simulink model "Angular_Input_Sliding_Mode"  (R2022a)
settings: Solver=VariableStepAuto  StartTime=0  StopTime=tspan(2)  RelTol=1e-8
undefined symbols (not defined in the file): Angle_max, b_Sxd, b_Syd, BL_gain, K_switch, lambda_x_num, r_sim, tau_angle, Tmax, x_0
libraries: cstblocks x4
settings Model: Creator=domin  LastModifiedBy=domin
settings SolverCC: AlgebraicLoopSolver=TrustRegion
settings DataIOCC: SaveFormat=StructureWithTime
settings OptimizationCC: BlockReduction=off  BufferReuse=off
settings DebuggingCC: AlgebraicLoopMsg=none  SFMachineParentedDataDiag=warning
settings RTWCC: DLArmComputeVersion=19.05

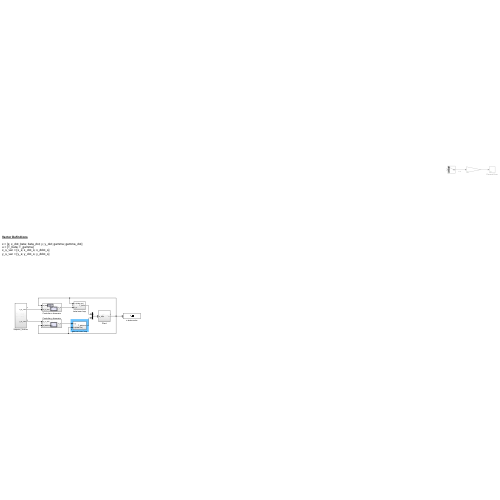
[thumbnail: Simulink's stored preview of the top-level diagram]
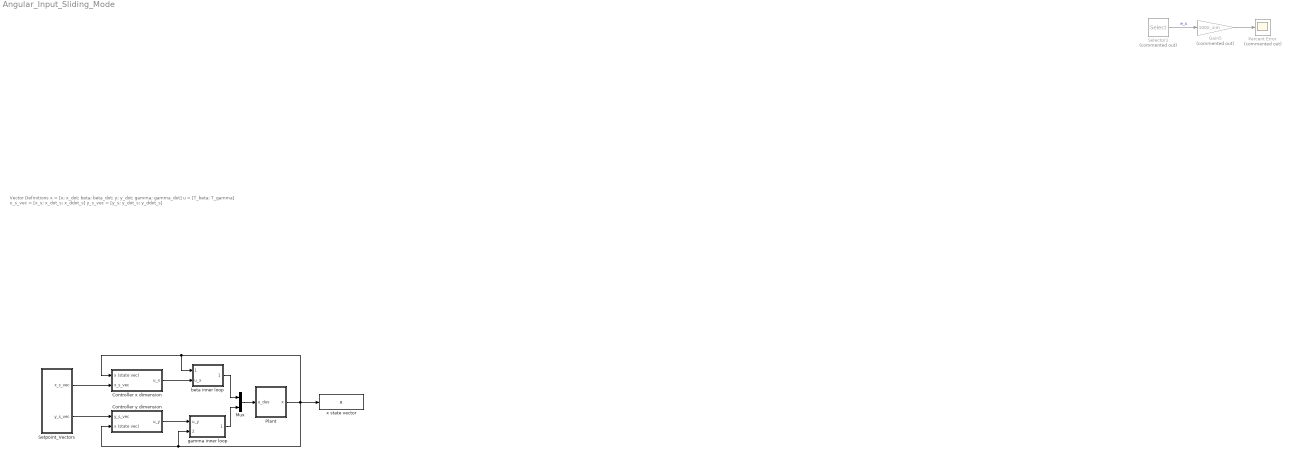
== system Angular_Input_Sliding_Mode ==
  note: Vector Definitions
      |
      | x = [x; x_dot; beta; beta_dot; y; y_dot; gamma; gamma_dot]
      | u = [T_beta; T_gamma]
      | x_s_vec = [x_s; x_dot_s; x_ddot_s]
      | y_s_vec = [y_s; y_dot_s; y_ddot_s]
  Controller x dimension : Subsystem
  Controller y dimension : Subsystem
  Gain5 : Gain  Commented=on  Gain=100/r_sim
  Mux : Mux  Inputs=2
  Percent Error : Scope  Commented=on
  Plant : Subsystem
  Selector1 : Selector  Commented=on  InputPortWidth=5  IndexOptions=Index vector (dialog)  Indices=[1]  OutputSizes=1
  Setpoint_Vectors : Subsystem
  beta inner loop : Subsystem
  gamma inner loop : Subsystem
  x state vector : ToWorkspace  VariableName=x  SampleTime=-1
  wires:
  Gain5/1 -> Percent Error/1
  Selector1/1 -> Gain5/1  "e_x"
  Controller x dimension/1(u_x) -> beta inner loop/2(u_x)
  Controller y dimension/1(u_y) -> gamma inner loop/1(u_y)
  Plant/1(x) -> Controller x dimension/1(x (state vec)), beta inner loop/1(x (state vec)), x state vector/1, Controller y dimension/2(x (state vec)), gamma inner loop/2(x (state vec))
  beta inner loop/1(T_beta) -> Mux/1
  Mux/1 -> Plant/1(u_des)
  gamma inner loop/1(T_gamma) -> Mux/2
  Setpoint_Vectors/1(x_s_vec) -> Controller x dimension/2(x_s_vec)
  Setpoint_Vectors/2(y_s_vec) -> Controller y dimension/1(y_s_vec)

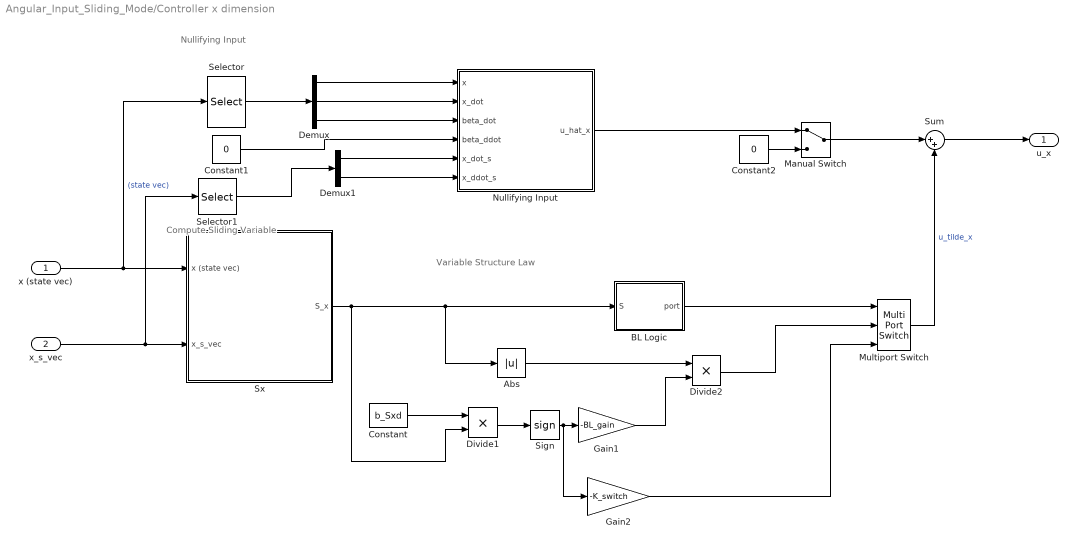
== system Angular_Input_Sliding_Mode/Controller x dimension ==
  note: Compute Sliding Variable
  note: Nullifying Input
  note: Variable Structure Law
  x (state vec) : Inport
  x_s_vec : Inport  Port=2
  Abs : Abs  SaturateOnIntegerOverflow=off
  BL Logic : MATLAB Function  TreatAsAtomicUnit=on
  Constant : Constant  Value=b_Sxd
  Constant1 : Constant  Value=0
  Constant2 : Constant  Value=0
  Demux : Demux  Outputs=3
  Demux1 : Demux  Outputs=2
  Divide1 : Product  Inputs=**
  Divide2 : Product  Inputs=**
  Gain1 : Gain  Gain=-BL_gain
  Gain2 : Gain  Gain=-K_switch
  Manual Switch : ManualSwitch
  Multiport Switch : MultiPortSwitch  Inputs=2  SaturateOnIntegerOverflow=off  InputSameDT=off
  Nullifying Input : MATLAB Function  TreatAsAtomicUnit=on
  Selector : Selector  InputPortWidth=8  IndexOptions=Index vector (dialog)  Indices=[1 2 4]  OutputSizes=1
  Selector1 : Selector  InputPortWidth=3  IndexOptions=Index vector (dialog)  Indices=[2 3]  OutputSizes=1
  Sign : Signum
  Sum : Sum  Inputs=|++
  Sx : Subsystem
  u_x : Outport
  wires:
  Sum/1 -> u_x/1
  x (state vec)/1 -> Sx/1(x (state vec)), Selector/1  "(state vec)"
  x_s_vec/1 -> Selector1/1, Sx/2(x_s_vec)
  Selector/1 -> Demux/1
  Demux/2 -> Nullifying Input/2(x_dot)
  Selector1/1 -> Demux1/1
  Demux1/1 -> Nullifying Input/5(x_dot_s)
  Demux1/2 -> Nullifying Input/6(x_ddot_s)
  Nullifying Input/1(u_hat_x) -> Manual Switch/1
  Constant/1 -> Divide1/1
  Divide2/1 -> Multiport Switch/2
  Sx/1(S_x) -> Divide1/2, Abs/1, BL Logic/1(S)
  Demux/1 -> Nullifying Input/1(x)
  Gain1/1 -> Divide2/2
  BL Logic/1(port) -> Multiport Switch/1
  Multiport Switch/1 -> Sum/2  "u_tilde_x"
  Sign/1 -> Gain2/1, Gain1/1
  Divide1/1 -> Sign/1
  Gain2/1 -> Multiport Switch/3
  Abs/1 -> Divide2/1
  Demux/3 -> Nullifying Input/3(beta_dot)
  Constant1/1 -> Nullifying Input/4(beta_ddot)
  Constant2/1 -> Manual Switch/2
  Manual Switch/1 -> Sum/1

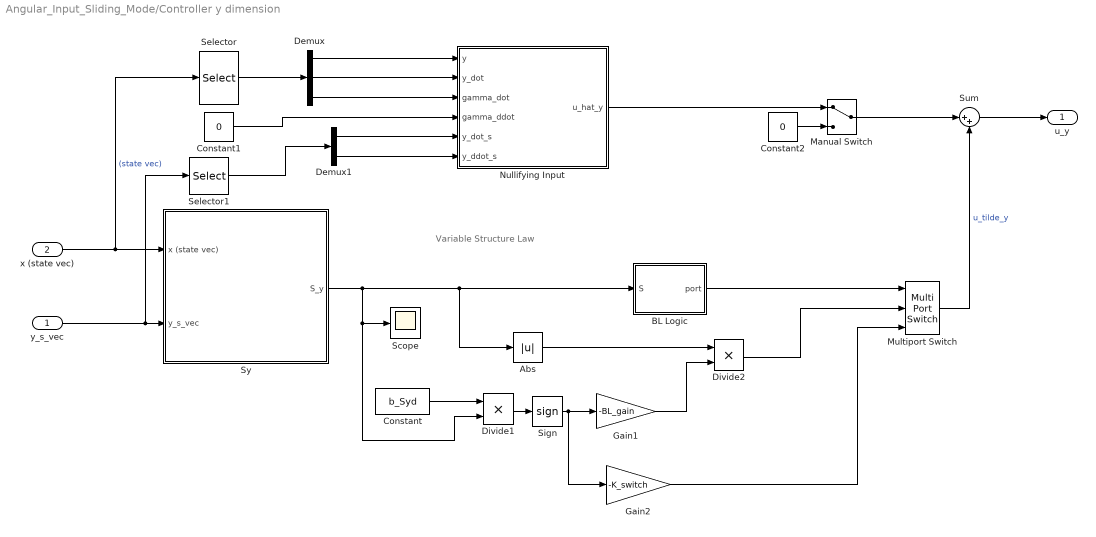
== system Angular_Input_Sliding_Mode/Controller y dimension ==
  note: Variable Structure Law
  y_s_vec : Inport
  x (state vec) : Inport  Port=2
  Abs : Abs  SaturateOnIntegerOverflow=off
  BL Logic : MATLAB Function  TreatAsAtomicUnit=on
  Constant : Constant  Value=b_Syd
  Constant1 : Constant  Value=0
  Constant2 : Constant  Value=0
  Demux : Demux  Outputs=3
  Demux1 : Demux  Outputs=2
  Divide1 : Product  Inputs=**
  Divide2 : Product  Inputs=**
  Gain1 : Gain  Gain=-BL_gain
  Gain2 : Gain  Gain=-K_switch
  Manual Switch : ManualSwitch
  Multiport Switch : MultiPortSwitch  Inputs=2  SaturateOnIntegerOverflow=off  InputSameDT=off
  Nullifying Input : MATLAB Function  TreatAsAtomicUnit=on
  Scope : Scope
  Selector : Selector  InputPortWidth=8  IndexOptions=Index vector (dialog)  Indices=[5 6 8]  OutputSizes=1
  Selector1 : Selector  InputPortWidth=3  IndexOptions=Index vector (dialog)  Indices=[2 3]  OutputSizes=1
  Sign : Signum
  Sum : Sum  Inputs=|++
  Sy : Subsystem
  u_y : Outport
  wires:
  Sum/1 -> u_y/1
  Gain1/1 -> Divide2/2
  Abs/1 -> Divide2/1
  Gain2/1 -> Multiport Switch/3
  Multiport Switch/1 -> Sum/2  "u_tilde_y"
  BL Logic/1(port) -> Multiport Switch/1
  Sign/1 -> Gain1/1, Gain2/1
  Constant/1 -> Divide1/1
  Divide2/1 -> Multiport Switch/2
  Sy/1(S_y) -> Divide1/2, Scope/1, Abs/1, BL Logic/1(S)
  Divide1/1 -> Sign/1
  Demux/3 -> Nullifying Input/3(gamma_dot)
  Demux/1 -> Nullifying Input/1(y)
  Demux1/1 -> Nullifying Input/5(y_dot_s)
  Nullifying Input/1(u_hat_y) -> Manual Switch/1
  Demux1/2 -> Nullifying Input/6(y_ddot_s)
  Selector/1 -> Demux/1
  Demux/2 -> Nullifying Input/2(y_dot)
  y_s_vec/1 -> Sy/2(y_s_vec), Selector1/1
  Selector1/1 -> Demux1/1
  x (state vec)/1 -> Sy/1(x (state vec)), Selector/1  "(state vec)"
  Constant1/1 -> Nullifying Input/4(gamma_ddot)
  Constant2/1 -> Manual Switch/2
  Manual Switch/1 -> Sum/1

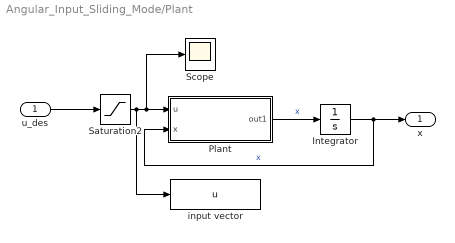
== system Angular_Input_Sliding_Mode/Plant ==
  u_des : Inport
  Integrator : Integrator  InitialCondition=x_0
  Plant : Subsystem
  Saturation2 : Saturate  UpperLimit=Tmax  LowerLimit=-Tmax  ZeroCross=off
  Scope : Scope
  input vector : ToWorkspace  VariableName=u  SampleTime=-1
  x : Outport
  wires:
  Saturation2/1 -> Scope/1, Plant/1(u), input vector/1
  Integrator/1 -> x/1, Plant/2(x)  "x"
  Plant/1(out1) -> Integrator/1  "x"
  u_des/1 -> Saturation2/1

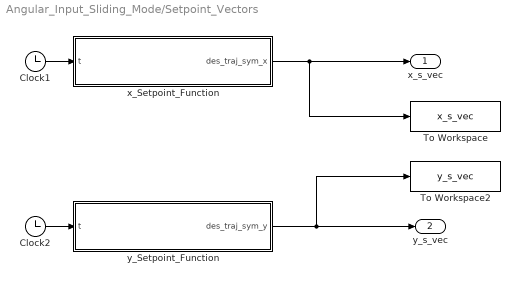
== system Angular_Input_Sliding_Mode/Setpoint_Vectors ==
  Clock1 : Clock
  Clock2 : Clock
  To Workspace : ToWorkspace  VariableName=x_s_vec  SampleTime=-1
  To Workspace2 : ToWorkspace  VariableName=y_s_vec  SampleTime=-1
  x_Setpoint_Function : MATLAB Function  TreatAsAtomicUnit=on
  y_Setpoint_Function : MATLAB Function  TreatAsAtomicUnit=on
  x_s_vec : Outport
  y_s_vec : Outport  Port=2
  wires:
  Clock2/1 -> y_Setpoint_Function/1(t)
  y_Setpoint_Function/1(des_traj_sym_y) -> y_s_vec/1, To Workspace2/1
  x_Setpoint_Function/1(des_traj_sym_x) -> x_s_vec/1, To Workspace/1
  Clock1/1 -> x_Setpoint_Function/1(t)

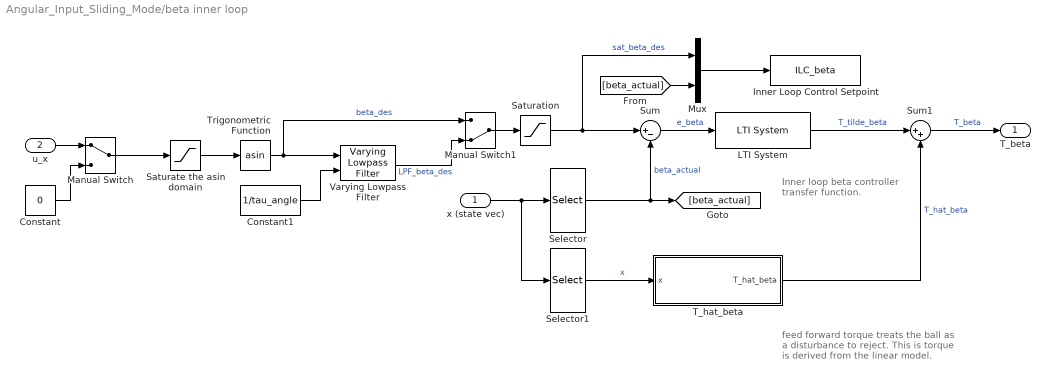
== system Angular_Input_Sliding_Mode/beta inner loop ==
  note: Inner loop beta controller
      | transfer function.
  note: feed forward torque treats the ball as a disturbance to reject. This is torque is derived from the linear model.
  x (state vec) : Inport
  u_x : Inport  Port=2
  Constant : Constant  Value=0
  Constant1 : Constant  Value=1/tau_angle
  Inner Loop Control Setpoint : ToWorkspace  VariableName=ILC_beta  SampleTime=-1
  LTI System : cstblocks/LTI System  sys=C_beta  IC=[]
  Manual Switch : ManualSwitch
  Manual Switch1 : ManualSwitch  CurrentSetting=0
  Mux : Mux  Inputs=2
  Saturate the asin domain : Saturate  UpperLimit=1  LowerLimit=-1
  Saturation : Saturate  UpperLimit=Angle_max  LowerLimit=-Angle_max
  Selector : Selector  InputPortWidth=8  IndexOptions=Index vector (dialog)  Indices=[3]  OutputSizes=1
  Selector1 : Selector  InputPortWidth=8  IndexOptions=Index vector (dialog)  Indices=[1]  OutputSizes=1
  Sum : Sum  Inputs=|+-
  Sum1 : Sum  Inputs=|++
  T_hat_beta : MATLAB Function  TreatAsAtomicUnit=on
  Trigonometric Function : Trigonometry  Operator=asin
  Varying Lowpass Filter : cstblocks/Linear Parameter Varying/Varying Lowpass Filter  N=1
  T_beta : Outport
  wires:
  u_x/1 -> Manual Switch/1
  Trigonometric Function/1 -> Manual Switch1/1, Varying Lowpass Filter/1  "beta_des"
  x (state vec)/1 -> Selector1/1, Selector/1
  Selector/1 -> Sum/2, [beta_actual]  "beta_actual"
  Sum/1 -> LTI System/1  "e_beta"
  Saturate the asin domain/1 -> Trigonometric Function/1
  LTI System/1 -> Sum1/1  "T_tilde_beta"
  T_hat_beta/1(T_hat_beta) -> Sum1/2  "T_hat_beta"
  Sum1/1 -> T_beta/1  "T_beta"
  Selector1/1 -> T_hat_beta/1(x)  "x"
  Constant/1 -> Manual Switch/2
  Manual Switch/1 -> Saturate the asin domain/1
  Constant1/1 -> Varying Lowpass Filter/2
  Varying Lowpass Filter/1 -> Manual Switch1/2  "LPF_beta_des"
  Mux/1 -> Inner Loop Control Setpoint/1
  Saturation/1 -> Sum/1, Mux/1  "sat_beta_des"
  Manual Switch1/1 -> Saturation/1
  [beta_actual] -> Mux/2

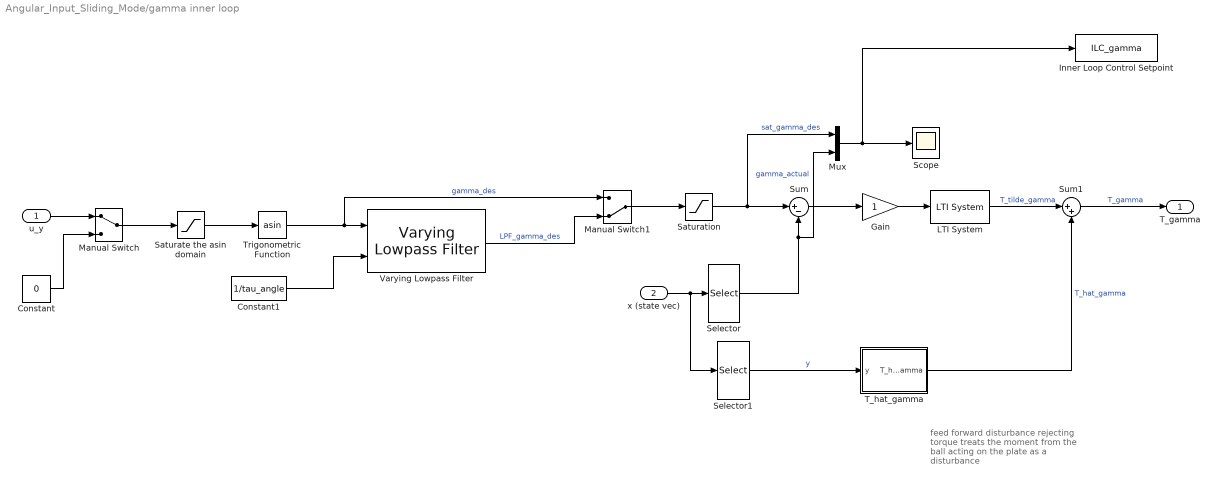
== system Angular_Input_Sliding_Mode/gamma inner loop ==
  note: feed forward disturbance rejecting torque treats the moment from the ball acting on the plate as a disturbance
  u_y : Inport
  x (state vec) : Inport  Port=2
  Constant : Constant  Value=0
  Constant1 : Constant  Value=1/tau_angle
  Gain : Gain
  Inner Loop Control Setpoint : ToWorkspace  VariableName=ILC_gamma  SampleTime=-1
  LTI System : cstblocks/LTI System  sys=C_gamma  IC=[]
  Manual Switch : ManualSwitch
  Manual Switch1 : ManualSwitch  CurrentSetting=0
  Mux : Mux  Inputs=2
  Saturate the asin domain : Saturate  UpperLimit=1  LowerLimit=-1
  Saturation : Saturate  UpperLimit=Angle_max  LowerLimit=-Angle_max
  Scope : Scope
  Selector : Selector  InputPortWidth=8  IndexOptions=Index vector (dialog)  Indices=[7]  OutputSizes=1
  Selector1 : Selector  InputPortWidth=8  IndexOptions=Index vector (dialog)  Indices=[5]  OutputSizes=1
  Sum : Sum  Inputs=|+-
  Sum1 : Sum  Inputs=|++
  T_hat_gamma : MATLAB Function  TreatAsAtomicUnit=on
  Trigonometric Function : Trigonometry  Operator=asin
  Varying Lowpass Filter : cstblocks/Linear Parameter Varying/Varying Lowpass Filter  N=1
  T_gamma : Outport
  wires:
  LTI System/1 -> Sum1/1  "T_tilde_gamma"
  Sum/1 -> Gain/1
  Selector/1 -> Mux/2, Sum/2  "gamma_actual"
  Trigonometric Function/1 -> Manual Switch1/1, Varying Lowpass Filter/1  "gamma_des"
  Saturation/1 -> Mux/1, Sum/1  "sat_gamma_des"
  Saturate the asin domain/1 -> Trigonometric Function/1
  T_hat_gamma/1(T_hat_gamma) -> Sum1/2  "T_hat_gamma"
  x (state vec)/1 -> Selector1/1, Selector/1
  Selector1/1 -> T_hat_gamma/1(y)  "y"
  Sum1/1 -> T_gamma/1  "T_gamma"
  u_y/1 -> Manual Switch/1
  Constant/1 -> Manual Switch/2
  Manual Switch/1 -> Saturate the asin domain/1
  Gain/1 -> LTI System/1
  Constant1/1 -> Varying Lowpass Filter/2
  Mux/1 -> Inner Loop Control Setpoint/1, Scope/1
  Varying Lowpass Filter/1 -> Manual Switch1/2  "LPF_gamma_des"
  Manual Switch1/1 -> Saturation/1

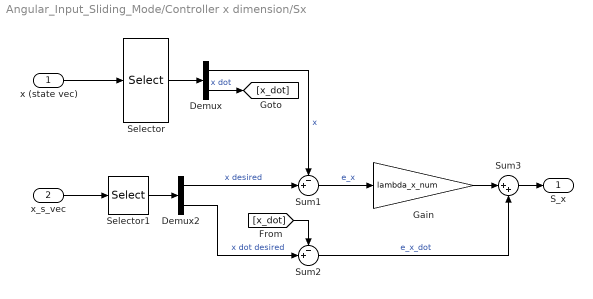
== system Angular_Input_Sliding_Mode/Controller x dimension/Sx ==
  x (state vec) : Inport
  x_s_vec : Inport  Port=2
  Demux : Demux  Outputs=2
  Demux2 : Demux  Outputs=2
  Gain : Gain  Gain=lambda_x_num
  Selector : Selector  InputPortWidth=8  IndexOptions=Index vector (dialog)  Indices=[1 2]  OutputSizes=1
  Selector1 : Selector  InputPortWidth=3  IndexOptions=Index vector (dialog)  Indices=[1 2]  OutputSizes=1
  Sum1 : Sum  Inputs=-+|
  Sum2 : Sum  Inputs=-+|
  Sum3 : Sum  Inputs=|++
  S_x : Outport
  wires:
  Demux/1 -> Sum1/1  "x"
  Demux2/2 -> Sum2/2  "x dot desired"
  Sum3/1 -> S_x/1
  x_s_vec/1 -> Selector1/1
  Selector1/1 -> Demux2/1
  Selector/1 -> Demux/1
  Sum2/1 -> Sum3/2  "e_x_dot"
  Demux/2 -> [x_dot]  "x dot"
  x (state vec)/1 -> Selector/1
  Demux2/1 -> Sum1/2  "x desired"
  Gain/1 -> Sum3/1
  Sum1/1 -> Gain/1  "e_x"
  [x_dot] -> Sum2/1

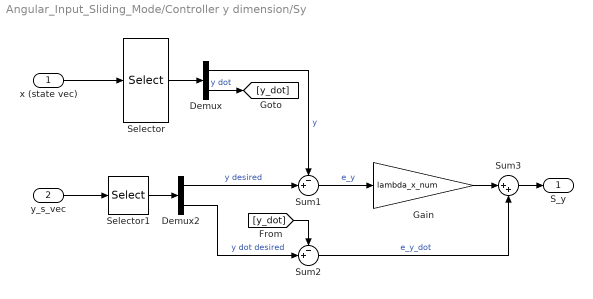
== system Angular_Input_Sliding_Mode/Controller y dimension/Sy ==
  x (state vec) : Inport
  y_s_vec : Inport  Port=2
  Demux : Demux  Outputs=2
  Demux2 : Demux  Outputs=2
  Gain : Gain  Gain=lambda_x_num
  Selector : Selector  InputPortWidth=8  IndexOptions=Index vector (dialog)  Indices=[5 6]  OutputSizes=1
  Selector1 : Selector  InputPortWidth=3  IndexOptions=Index vector (dialog)  Indices=[1 2]  OutputSizes=1
  Sum1 : Sum  Inputs=-+|
  Sum2 : Sum  Inputs=-+|
  Sum3 : Sum  Inputs=|++
  S_y : Outport
  wires:
  Demux/2 -> [y_dot]  "y dot"
  [y_dot] -> Sum2/1
  Gain/1 -> Sum3/1
  Demux2/1 -> Sum1/2  "y desired"
  Selector/1 -> Demux/1
  Sum2/1 -> Sum3/2  "e_y_dot"
  x (state vec)/1 -> Selector/1
  y_s_vec/1 -> Selector1/1
  Sum3/1 -> S_y/1
  Selector1/1 -> Demux2/1
  Demux2/2 -> Sum2/2  "y dot desired"
  Sum1/1 -> Gain/1  "e_y"
  Demux/1 -> Sum1/1  "y"

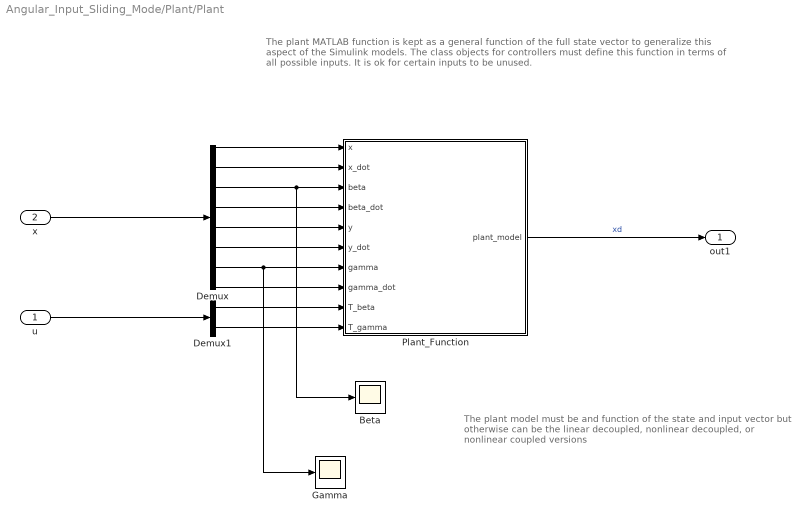
== system Angular_Input_Sliding_Mode/Plant/Plant ==
  note: The plant MATLAB function is kept as a general function of the full state vector
      | to generalize this aspect of the Simulink models. The class objects for controllers must define this function in terms of all possible inputs. It is ok for certain inputs to be unused.
  note: The plant model must be and function of the state and input vector
      |  but otherwise can be the linear decoupled, nonlinear decoupled,
      | or nonlinear coupled versions
  u : Inport
  x : Inport  Port=2
  Beta : Scope
  Demux : Demux  Outputs=8
  Demux1 : Demux  Outputs=2
  Gamma : Scope
  Plant_Function : MATLAB Function  TreatAsAtomicUnit=on
  out1 : Outport
  wires:
  Demux1/1 -> Plant_Function/9(T_beta)
  Demux1/2 -> Plant_Function/10(T_gamma)
  Demux/5 -> Plant_Function/5(y)
  Demux/8 -> Plant_Function/8(gamma_dot)
  Demux/1 -> Plant_Function/1(x)
  Demux/3 -> Beta/1, Plant_Function/3(beta)
  Demux/4 -> Plant_Function/4(beta_dot)
  Demux/2 -> Plant_Function/2(x_dot)
  Demux/6 -> Plant_Function/6(y_dot)
  x/1 -> Demux/1
  Plant_Function/1(plant_model) -> out1/1  "xd"
  u/1 -> Demux1/1
  Demux/7 -> Gamma/1, Plant_Function/7(gamma)

== matlab function Angular_Input_Sliding_Mode/Plant/Plant/Plant_Function ==
  data: x input; plant_model output size=8; x_dot input; beta input; beta_dot input; y input; y_dot input; gamma input; gamma_dot input; T_beta input; T_gamma input
function plant_model = xdot(x,x_dot,beta,beta_dot,y,y_dot,gamma,gamma_dot,T_beta,T_gamma)
%#codegen

%    This function was generated by the Symbolic Math Toolbox version 9.1.
%    03-Nov-2022 15:11:18

t2 = cos(beta);
t3 = cos(gamma);
t4 = sin(beta);
t5 = sin(gamma);
t6 = beta_dot.^2;
t7 = gamma_dot.^2;
t8 = x.^2;
t9 = x.^3;
t10 = y.^2;
t11 = y.^3;
t13 = y.^5;
t12 = t10.^2;
t14 = t3.^2;
t15 = t3.^3;
t17 = t3.^5;
t19 = t5.^2;
t20 = t5.^3;
t22 = t5.^5;
t29 = t3.*t5.*t8.*y.*6.9103125e-2;
t35 = t3.*t5.*y.*2.54656384453125e-1;
t16 = t14.^2;
t18 = t14.^3;
t21 = t19.^2;
t24 = t8.*t19.*1.24425;
t26 = t12.*t14.*t19.*(5.67e+2./1.6e+2);
t27 = t3.*t11.*t20.*7.2646875e-1;
t28 = t5.*t11.*t15.*7.2646875e-1;
t30 = -t29;
t31 = t8.*t10.*t14.*t19.*(5.67e+2./1.6e+2);
t32 = t3.*t8.*t20.*y.*7.95571875e-1;
t33 = t5.*t8.*t15.*y.*7.95571875e-1;
t34 = t10.*t19.*1.242226265625;
t36 = t8.*t14.*4.3477919296875;
t37 = t19.*6.612991525054688e-4;
t42 = t3.*t20.*y.*9.706520554870837e-2;
t43 = t5.*t15.*y.*9.706520554870837e-2;
t44 = t10.*t14.*t19.*6.480378078996037;
t45 = t8.*t14.*t19.*2.118038321496037;
t47 = t14.*2.104993904427172;
t49 = t14.*t19.*8.025946633503326e-1;
t23 = t12.*t21.*(5.67e+2./1.6e+2);
t25 = t8.*t10.*t21.*(5.67e+2./1.6e+2);
t38 = t8.*t21.*4.60827495054675e-1;
t39 = t10.*t21.*4.75375322867175e-1;
t40 = t10.*t16.*6.005002756128863;
t41 = t8.*t16.*1.657210826441363;
t46 = t21.*2.520617667017312e-4;
t48 = t16.*8.023426015836309e-1;
t50 = t23+t24+t25+t26+t27+t28+t30+t31+t32+t33+t34+t35+t36+t37+t38+t39+t40+t41+t42+t43+t44+t45+t46+t47+t48+t49;
t51 = 1.0./t50;
et1 = T_beta.*t3.*(-1.7915663253125)-T_beta.*t15.*6.828760802288535e-1+t4.*t14.*8.635902280667424+t4.*t16.*3.291673333742159;
et2 = t4.*t19.*4.63381763291332e-3+t4.*t21.*1.766232808102845e-3-T_beta.*t3.*t19.*6.828760802288535e-1-T_beta.*t10.*t15.*5.110875-T_beta.*t11.*t20.*(3.15e+2./8.0)+beta_dot.*gamma_dot.*t20.*1.189393761434836e-4;
et3 = beta_dot.*gamma_dot.*t22.*4.533510918249709e-5-T_beta.*t5.*y.*1.38025140625e+1-T_beta.*t20.*y.*5.2609867506075-beta_dot.*t20.*y_dot.*1.133655690009375e-3-beta_dot.*t22.*y_dot.*4.321058857743964e-4;
et4 = t4.*t8.*t14.*3.046559916445312e+1+t4.*t8.*t16.*1.16123130052784e+1+t6.*t9.*t14.*3.1055656640625+t4.*t10.*t16.*2.463599390383014e+1+t4.*t8.*t19.*8.7186375+t6.*t9.*t16.*1.183722018886688;
et5 = t4.*t8.*t21.*3.229084090347401+t6.*t9.*t19.*(7.11e+2./8.0e+2)+t4.*t10.*t21.*1.3219082296875e-2+t6.*t9.*t21.*3.29162496467625e-1+t4.*t14.*t19.*3.293439566550262;
et6 = t2.*t3.*x.*(-3.954434771546016)-t2.*t15.*x.*1.507278228085137+t6.*t14.*x.*1.49176193219726+t7.*t14.*x.*4.917849562982812e-2;
et7 = t6.*t16.*x.*6.177806883037708e-1+t7.*t16.*x.*1.874494840228203e-2+t6.*t18.*x.*1.874494840228203e-2+t6.*t19.*x.*4.723565375039063e-4;
et8 = t6.*t21.*x.*1.800441190726652e-4-T_beta.*t5.*t11.*t14.*(3.15e+2./8.0)-T_beta.*t3.*t10.*t19.*5.110875-beta_dot.*gamma_dot.*t5.*t14.*1.189671157991527e-2-beta_dot.*gamma_dot.*t5.*t16.*4.534568247083289e-3;
et9 = beta_dot.*gamma_dot.*t8.*t20.*2.2378725e-1-beta_dot.*gamma_dot.*t11.*t17.*8.511221334648375+beta_dot.*gamma_dot.*t8.*t22.*8.288311661054797e-2+beta_dot.*gamma_dot.*t10.*t20.*2.42234121796875e-2+beta_dot.*gamma_dot.*t10.*t22.*9.572335001378663e-3+beta_dot.*gamma_dot.*t12.*t22.*6.9103125e-2;
et10 = beta_dot.*gamma_dot.*t14.*t20.*(-4.489233137900792e-3)+T_gamma.*t3.*t5.*x.*1.49675625e-1-T_beta.*t5.*t14.*y.*5.2609867506075-beta_dot.*gamma_dot.*t15.*y.*2.98352386439452;
et11 = beta_dot.*gamma_dot.*t17.*y.*(-1.137204385347885)-T_gamma.*t14.*x.*y.*5.110875+T_gamma.*t19.*x.*y.*(3.69e+2./3.2e+2)-beta_dot.*t5.*t14.*y_dot.*3.599900035525355-beta_dot.*t5.*t16.*y_dot.*1.372143241778375;
et12 = beta_dot.*t8.*t20.*y_dot.*(-2.133)-beta_dot.*t8.*t22.*y_dot.*7.899899915223e-1-beta_dot.*t10.*t20.*y_dot.*1.242226265625-beta_dot.*t10.*t22.*y_dot.*4.76722833804675e-1-beta_dot.*t12.*t22.*y_dot.*(5.67e+2./1.6e+2)-beta_dot.*t14.*t20.*y_dot.*1.37257534766415;
et13 = beta_dot.*t15.*x.*x_dot.*8.06204846390625e-1+beta_dot.*t17.*x.*x_dot.*3.072942361029841e-1-gamma_dot.*t3.*t5.*x_dot.*3.144198900923438e-3-gamma_dot.*t5.*t15.*x_dot.*1.198447520801638e-3-gamma_dot.*t3.*t20.*x_dot.*1.198447520801638e-3;
et14 = gamma_dot.*t11.*t21.*x_dot.*(-6.9103125e-2)-gamma_dot.*t14.*x.*y_dot.*8.06204846390625e-1-gamma_dot.*t16.*x.*y_dot.*3.072942361029841e-1-gamma_dot.*t19.*x_dot.*y.*2.42234121796875e-2-gamma_dot.*t21.*x_dot.*y.*9.233031747316162e-3-t4.*t5.*t11.*t15.*1.325079998274375e+2;
et15 = t3.*t4.*t11.*t20.*(-1.325079998274375e+2)+t4.*t8.*t10.*t21.*2.48315625e+1+t4.*t8.*t14.*t19.*1.484139709562581e+1+t6.*t9.*t10.*t21.*(8.1e+1./3.2e+1)+t4.*t10.*t14.*t19.*2.464921298612702e+1+t6.*t9.*t14.*t19.*1.512884515354313;
et16 = t2.*t3.*t19.*x.*1.85690659069221+t2.*t3.*t21.*x.*1.047837787317732-t6.*t10.*t14.*x.*6.406846875e-3-t7.*t10.*t14.*x.*6.406846875e-3+t6.*t10.*t16.*x.*4.302101376699188-t2.*t11.*t20.*x.*8.691046875e+1;
et17 = t7.*t10.*t16.*x.*4.00838625e-2-t6.*t10.*t18.*x.*4.00838625e-2+t2.*t11.*t22.*x.*6.207890625e+1+t6.*t10.*t19.*x.*(7.11e+2./8.0e+2)+t2.*t15.*t19.*x.*1.047837787317732+t7.*t10.*t19.*x.*(7.11e+2./8.0e+2)+t6.*t10.*t21.*x.*3.30510007405125e-1+t7.*t10.*t21.*x.*3.60815777717625e-1;
et18 = t6.*t12.*t21.*x.*(8.1e+1./3.2e+1)+t6.*t14.*t19.*x.*5.710317519180153e-1+t7.*t12.*t21.*x.*(8.1e+1./3.2e+1)+t7.*t14.*t19.*x.*1.874494840228203e-2+t6.*t14.*t21.*x.*8.331431948092056e-4;
et19 = t6.*t16.*t19.*x.*1.957809159709123e-2-t3.*t4.*t5.*y.*4.64493595177639e+1-t4.*t5.*t15.*y.*1.770470683026412e+1-t3.*t4.*t20.*y.*1.770470683026412e+1;
et20 = t2.*t5.*x.*y.*(-3.046559916445312e+1)+t2.*t20.*x.*y.*1.430590593753628e+1+t2.*t22.*x.*y.*8.072710225868503+beta_dot.*gamma_dot.*t5.*t8.*t14.*7.819814342109375e-1+beta_dot.*gamma_dot.*t5.*t8.*t16.*2.980612043556679e-1;
et21 = beta_dot.*gamma_dot.*t5.*t10.*t14.*4.8446824359375e-2-beta_dot.*gamma_dot.*t5.*t10.*t16.*1.547217531737134e-2+beta_dot.*gamma_dot.*t5.*t12.*t16.*1.3820625e-1-beta_dot.*gamma_dot.*t3.*t11.*t21.*8.528082497148375+beta_dot.*gamma_dot.*t8.*t10.*t22.*6.3736875e-1+beta_dot.*gamma_dot.*t8.*t14.*t20.*3.809443209662159e-1;
et22 = beta_dot.*gamma_dot.*t10.*t14.*t20.*(-5.899840315992675e-3)-beta_dot.*gamma_dot.*t11.*t15.*t19.*1.703930383179675e+1+beta_dot.*gamma_dot.*t12.*t14.*t20.*2.07309375e-1-T_gamma.*t3.*t5.*t10.*x.*(3.15e+2./8.0)-beta_dot.*gamma_dot.*t3.*t19.*y.*2.989434376966363-beta_dot.*gamma_dot.*t8.*t15.*y.*6.211131328125;
et23 = beta_dot.*gamma_dot.*t3.*t21.*y.*(-1.13945724509423)-beta_dot.*gamma_dot.*t8.*t17.*y.*2.367444037773375-beta_dot.*gamma_dot.*t15.*t19.*y.*2.276661630442116-beta_dot.*t5.*t8.*t14.*y_dot.*7.45335759375;
et24 = beta_dot.*t5.*t8.*t16.*y_dot.*(-2.84093284532805)-beta_dot.*t5.*t10.*t16.*y_dot.*1.026958300907805e+1-beta_dot.*t3.*t11.*t21.*y_dot.*7.2646875e-1-beta_dot.*t8.*t10.*t22.*y_dot.*(2.43e+2./4.0e+1)-beta_dot.*t8.*t14.*t20.*y_dot.*3.63092283685035-beta_dot.*t10.*t14.*t20.*y_dot.*1.074630584288272e+1-beta_dot.*t11.*t15.*t19.*y_dot.*7.2646875e-1;
et25 = beta_dot.*t12.*t14.*t20.*y_dot.*(-5.67e+2./1.6e+2)+beta_dot.*t3.*t19.*x.*x_dot.*1.1535975e-1+beta_dot.*t3.*t21.*x.*x_dot.*4.272529204149773e-2+beta_dot.*t11.*t22.*x.*x_dot.*(8.1e+1./3.2e+1)+beta_dot.*t15.*t19.*x.*x_dot.*3.500195281444818e-1-gamma_dot.*t5.*t10.*t15.*x_dot.*8.969585625e-3-gamma_dot.*t3.*t10.*t20.*x_dot.*8.969585625e-3-gamma_dot.*t11.*t14.*t19.*x_dot.*6.9103125e-2;
et26 = beta_dot.*t3.*t19.*y.*y_dot.*(-2.54656384453125e-1)-beta_dot.*t3.*t21.*y.*y_dot.*9.706520554870837e-2-beta_dot.*t15.*t19.*y.*y_dot.*9.706520554870837e-2+beta_dot.*t20.*x.*x_dot.*y.*(7.11e+2./8.0e+2)+beta_dot.*t22.*x.*x_dot.*y.*3.29162496467625e-1-gamma_dot.*t10.*t21.*x.*y_dot.*5.1890625e-1;
et27 = gamma_dot.*t14.*t19.*x.*y_dot.*(-3.072942361029841e-1)-gamma_dot.*t14.*t19.*x_dot.*y.*9.233031747316162e-3+t4.*t8.*t10.*t14.*t19.*2.48315625e+1+t6.*t9.*t10.*t14.*t19.*(8.1e+1./3.2e+1)-t3.*t5.*t6.*t11.*x.*4.9359375e-2-t3.*t5.*t7.*t11.*x.*4.9359375e-2-t2.*t3.*t10.*t19.*x.*1.557751738899375e+2;
et28 = t2.*t3.*t10.*t21.*x.*1.563146859375e+1+t5.*t6.*t11.*t15.*x.*6.17625e-1+t5.*t7.*t11.*t15.*x.*6.3736875e-1-t5.*t6.*t11.*t17.*x.*6.3736875e-1+t3.*t6.*t11.*t20.*x.*5.68265625e-1+t3.*t7.*t11.*t20.*x.*6.3736875e-1+t3.*t6.*t11.*t22.*x.*5.68265625e-1+t2.*t10.*t15.*t19.*x.*1.563146859375e+1+t2.*t11.*t14.*t20.*x.*6.207890625e+1;
et29 = t6.*t10.*t14.*t19.*x.*9.947623357541812+t7.*t10.*t14.*t19.*x.*4.00899640217625e-1+t6.*t10.*t14.*t21.*x.*2.14971754443075+t6.*t10.*t16.*t19.*x.*2.10963368193075+t6.*t12.*t14.*t19.*x.*(8.1e+1./3.2e+1)-t6.*t11.*t15.*t20.*x.*6.9103125e-2+t7.*t12.*t14.*t19.*x.*(8.1e+1./3.2e+1)-t6.*t12.*t14.*t21.*x.*(8.1e+1./3.2e+1);
et30 = t6.*t12.*t16.*t19.*x.*(-8.1e+1./3.2e+1)-t3.*t4.*t5.*t8.*y.*4.8421546875e-1-t3.*t5.*t6.*t9.*y.*4.9359375e-2+t4.*t5.*t8.*t15.*y.*5.57468578125+t3.*t4.*t8.*t20.*y.*5.57468578125+t5.*t6.*t9.*t15.*y.*5.68265625e-1+t3.*t6.*t9.*t20.*y.*5.68265625e-1+t3.*t5.*t6.*x.*y.*9.11363378203125e-2+t3.*t5.*t7.*x.*y.*4.94238761015625e-1;
et31 = t2.*t5.*t14.*x.*y.*(-3.036765952227354e+1)+t2.*t5.*t16.*x.*y.*9.830567278125e-1+t5.*t6.*t15.*x.*y.*1.103091434186369+t5.*t7.*t15.*x.*y.*1.912479742519236e-1+t5.*t6.*t17.*x.*y.*4.138732615906622e-1;
et32 = t3.*t6.*t20.*x.*y.*5.082288529418156e-2+t3.*t7.*t20.*x.*y.*1.912479742519236e-1+t3.*t6.*t22.*x.*y.*6.418668681118688e-3+t2.*t14.*t20.*x.*y.*9.055766953681003+t6.*t15.*t20.*x.*y.*4.202919302717809e-1;
et33 = beta_dot.*t8.*t10.*t14.*t20.*y_dot.*(-2.43e+2./4.0e+1)-beta_dot.*t3.*t10.*t19.*x.*x_dot.*4.9359375e-2+beta_dot.*t3.*t10.*t21.*x.*x_dot.*1.156275+beta_dot.*t10.*t15.*t19.*x.*x_dot.*1.156275+beta_dot.*t11.*t14.*t20.*x.*x_dot.*(8.1e+1./3.2e+1)+beta_dot.*t3.*t8.*t19.*y.*y_dot.*1.184625e-1-beta_dot.*t3.*t8.*t21.*y.*y_dot.*1.3638375-beta_dot.*t8.*t15.*t19.*y.*y_dot.*1.3638375+beta_dot.*t5.*t14.*x.*x_dot.*y.*6.20472448125;
et34 = beta_dot.*t5.*t16.*x.*x_dot.*y.*2.474881931523375+beta_dot.*t14.*t20.*x.*x_dot.*y.*2.804044427991-gamma_dot.*t10.*t14.*t19.*x.*y_dot.*5.1890625e-1-gamma_dot.*t3.*t5.*x.*y.*y_dot.*6.211131328125-gamma_dot.*t5.*t15.*x.*y.*y_dot.*2.434798069023375-gamma_dot.*t3.*t20.*x.*y.*y_dot.*2.434798069023375;
et35 = beta_dot.*gamma_dot.*t5.*t8.*t10.*t14.*9.871875e-2-beta_dot.*gamma_dot.*t5.*t8.*t10.*t16.*1.13653125-beta_dot.*gamma_dot.*t3.*t8.*t11.*t21.*(8.1e+1./1.6e+1)-beta_dot.*gamma_dot.*t8.*t10.*t14.*t20.*4.991625e-1-beta_dot.*gamma_dot.*t8.*t11.*t15.*t19.*(8.1e+1./1.6e+1)-beta_dot.*gamma_dot.*t3.*t8.*t19.*y.*1.789928690625-beta_dot.*gamma_dot.*t3.*t8.*t21.*y.*5.1523570856025e-1-beta_dot.*gamma_dot.*t8.*t15.*t19.*y.*2.882679746333625;
et36 = T_beta.*(-1.93235196875e+1)-T_beta.*t14.*7.3653814508505-T_beta.*t19.*7.3653814508505-t3.*t4.*6.594550854773621e+1-t4.*t15.*2.513588793756854e+1;
et37 = t2.*x.*(-4.265183883023438e+1)-T_beta.*t10.*t14.*(4.41e+2./8.0)-T_beta.*t10.*t19.*(4.41e+2./8.0)+T_gamma.*t5.*x.*1.614375-gamma_dot.*t5.*x_dot.*3.39127770515625e-2-gamma_dot.*t20.*x_dot.*1.292624444624263e-2-t3.*t4.*t19.*2.513588793756854e+1;
et38 = t4.*t10.*t15.*(-1.881254666584125e+2)-t4.*t11.*t20.*3.47641875e+1-t3.*t6.*x.*1.273281922265625e-1+t3.*t7.*x.*5.30430615421875e-1-t2.*t14.*x.*1.625723820738977e+1+t2.*t19.*x.*2.00282683125508e+1;
et39 = t6.*t15.*x.*4.818980126475208e-1+t7.*t15.*x.*2.021797208258462e-1+t2.*t21.*x.*1.13017943162159e+1+t6.*t17.*x.*2.021797208258462e-1-t4.*t5.*y.*1.218623966578125e+1;
et40 = t4.*t20.*y.*(-4.644925202111362)-beta_dot.*gamma_dot.*t3.*t5.*4.211809409450256-beta_dot.*gamma_dot.*t5.*t15.*1.60537952715466;
et41 = beta_dot.*gamma_dot.*t3.*t20.*(-1.60537952715466)+beta_dot.*gamma_dot.*t11.*t16.*7.2646875e-1-beta_dot.*gamma_dot.*t11.*t21.*7.95571875e-1+beta_dot.*gamma_dot.*t14.*y.*2.54656384453125e-1+beta_dot.*gamma_dot.*t16.*y.*9.706520554870837e-2-beta_dot.*gamma_dot.*t19.*y.*2.788797966328125e-1;
et42 = beta_dot.*gamma_dot.*t21.*y.*(-1.062982372960245e-1)-T_gamma.*t3.*x.*y.*(4.41e+2./8.0)+beta_dot.*t3.*t5.*y_dot.*9.3415415175e-2+beta_dot.*t5.*t15.*y_dot.*3.560635832811156e-2+beta_dot.*t3.*t20.*y_dot.*3.560635832811156e-2+beta_dot.*t11.*t21.*y_dot.*(5.67e+2./1.6e+2)+beta_dot.*t14.*x.*x_dot.*8.695583859375;
et43 = beta_dot.*t16.*x.*x_dot.*3.314421652882725+beta_dot.*t19.*x.*x_dot.*1.24425+beta_dot.*t21.*x.*x_dot.*4.60827495054675e-1-gamma_dot.*t5.*t14.*x_dot.*1.292624444624263e-2-gamma_dot.*t10.*t20.*x_dot.*9.6744375e-2+beta_dot.*t19.*y.*y_dot.*1.242226265625;
et44 = beta_dot.*t21.*y.*y_dot.*4.73488807554675e-1-gamma_dot.*t3.*x.*y_dot.*8.695583859375-gamma_dot.*t15.*x.*y_dot.*3.314421652882725-t4.*t5.*t11.*t14.*3.47641875e+1-t3.*t4.*t10.*t19.*1.881254666584125e+2-t3.*t6.*t10.*x.*6.9103125e-2-t3.*t7.*t10.*x.*6.9103125e-2;
et45 = t3.*t6.*t19.*x.*(-2.426972777435419e-2)+t3.*t7.*t19.*x.*2.021797208258462e-1+t3.*t6.*t21.*x.*8.986136153566162e-3-t2.*t10.*t19.*x.*1.2167465625e+2+t6.*t10.*t15.*x.*1.3820625e-1+t7.*t10.*t15.*x.*4.323375e-1+t2.*t10.*t21.*x.*8.691046875e+1;
et46 = t6.*t10.*t17.*x.*(-4.323375e-1)+t2.*t14.*t19.*x.*1.13017943162159e+1+t7.*t11.*t20.*x.*(5.67e+2./1.6e+2)+t6.*t15.*t19.*x.*2.111658569794124e-1-t4.*t5.*t14.*y.*4.644925202111362+t5.*t6.*x.*y.*2.023734375e-3+t5.*t7.*x.*y.*1.24425;
et47 = t6.*t20.*x.*y.*(-1.26613125e-2)+t7.*t20.*x.*y.*5.05142088804675e-1+beta_dot.*gamma_dot.*t3.*t5.*t10.*2.48445253125-beta_dot.*gamma_dot.*t5.*t10.*t15.*1.106822445214838e+1+beta_dot.*gamma_dot.*t5.*t12.*t15.*(5.67e+2./8.0e+1)-beta_dot.*gamma_dot.*t3.*t10.*t20.*1.106822445214838e+1+beta_dot.*gamma_dot.*t3.*t12.*t20.*(5.67e+2./8.0e+1)-beta_dot.*gamma_dot.*t11.*t14.*t19.*6.9103125e-2;
et48 = beta_dot.*gamma_dot.*t14.*t19.*y.*(-9.233031747316162e-3)+beta_dot.*t5.*t10.*t15.*y_dot.*2.6649e-1+beta_dot.*t3.*t10.*t20.*y_dot.*2.6649e-1+beta_dot.*t11.*t14.*t19.*y_dot.*(5.67e+2./1.6e+2)+beta_dot.*t10.*t21.*x.*x_dot.*(5.67e+2./1.6e+2)+beta_dot.*t14.*t19.*x.*x_dot.*3.7752491479374-gamma_dot.*t5.*t10.*t14.*x_dot.*9.6744375e-2+beta_dot.*t14.*t19.*y.*y_dot.*4.73488807554675e-1;
et49 = gamma_dot.*t3.*t19.*x.*y_dot.*(-3.314421652882725)-gamma_dot.*t20.*x.*y.*y_dot.*7.2646875e-1+t5.*t7.*t11.*t14.*x.*(5.67e+2./1.6e+2)+t3.*t6.*t10.*t19.*x.*6.9103125e-2-t5.*t6.*t11.*t16.*x.*(5.67e+2./1.6e+2)+t3.*t7.*t10.*t19.*x.*4.323375e-1+t3.*t6.*t10.*t21.*x.*7.95571875e-1+t2.*t10.*t14.*t19.*x.*8.691046875e+1+t6.*t10.*t15.*t19.*x.*3.63234375e-1-t6.*t11.*t14.*t20.*x.*(5.67e+2./1.6e+2);
et50 = t2.*t3.*t5.*x.*y.*(-2.022918730646625e+2)+t2.*t5.*t15.*x.*y.*1.06030771875e+1+t2.*t3.*t20.*x.*y.*1.06030771875e+1+t5.*t6.*t14.*x.*y.*7.4373250359375+t5.*t7.*t14.*x.*y.*5.05142088804675e-1+t5.*t6.*t16.*x.*y.*2.90633933282805;
et51 = t6.*t14.*t20.*x.*y.*2.90633933282805+beta_dot.*t10.*t14.*t19.*x.*x_dot.*(5.67e+2./1.6e+2)-beta_dot.*t3.*t5.*x.*x_dot.*y.*6.9103125e-2+beta_dot.*t5.*t15.*x.*x_dot.*y.*1.15880625+beta_dot.*t3.*t20.*x.*x_dot.*y.*1.15880625-gamma_dot.*t5.*t14.*x.*y.*y_dot.*7.2646875e-1;
et52 = T_gamma.*t14.*2.474442405541354+T_gamma.*t19.*7.773640875e-4-t2.*t20.*1.831378936369438e-3-t2.*t22.*1.915755736403127e-3+T_gamma.*t8.*t14.*5.110875+T_gamma.*t8.*t19.*3.07125e-1+T_gamma.*t10.*t19.*1.46025;
et53 = T_beta.*t5.*x.*1.38309889375e+1+T_beta.*t20.*x.*5.0828362506075+beta_dot.*t20.*x_dot.*1.134630171419062e-3+beta_dot.*t22.*x_dot.*4.260091302881464e-4+t2.*t5.*t8.*3.052845033229687e+1;
et54 = t2.*t5.*t14.*(-5.829497109059283)-t2.*t5.*t16.*6.0980785053503-t5.*t6.*t15.*1.16673363209345e-2;
et55 = t5.*t6.*t17.*(-4.8486251112877e-3)-t3.*t6.*t20.*3.665378605041563e-6-t2.*t8.*t20.*1.819838125034571e+1-t3.*t6.*t22.*1.523230860748663e-6;
et56 = t2.*t8.*t22.*(-1.13017943162159e+1)-t2.*t10.*t20.*3.440178334496925+t6.*t11.*t16.*4.289287682949187-t2.*t10.*t22.*3.611896148894276+t7.*t11.*t16.*4.289287682949187;
et57 = t6.*t11.*t18.*(-4.289287682949187)-t2.*t12.*t22.*2.48315625e+1-t2.*t14.*t20.*6.099994261086703+t6.*t11.*t19.*8.89135003125e-1+t7.*t11.*t19.*8.89135003125e-1+t6.*t11.*t21.*3.28101269905125e-1;
et58 = t7.*t11.*t21.*3.68185132405125e-1+t6.*t13.*t21.*(8.1e+1./3.2e+1)-t6.*t15.*t20.*4.850148342148449e-3+t7.*t13.*t21.*(8.1e+1./3.2e+1)-t2.*t15.*y.*5.461712999631153;
et59 = t6.*t14.*y.*1.506668964892069+t7.*t14.*y.*1.506668964892069-t6.*t16.*y.*9.529738049129356e-1;
et60 = t7.*t16.*y.*6.216186040112436e-1-t6.*t18.*y.*4.857717159470233e-1+t6.*t19.*y.*4.733310189135937e-4+t7.*t19.*y.*4.733310189135937e-4;
et61 = t6.*t21.*y.*1.739473635864152e-4+t7.*t21.*y.*1.952860077882902e-4+T_beta.*t5.*t14.*x.*5.0828362506075+T_beta.*t10.*t20.*x.*(3.15e+2./8.0)+T_gamma.*t3.*t5.*y.*2.9935125e-1+T_beta.*t15.*x.*y.*5.110875;
et62 = beta_dot.*t5.*t14.*x_dot.*3.611662869319241+beta_dot.*t5.*t16.*x_dot.*1.356037761562764+beta_dot.*t8.*t20.*x_dot.*1.24425+beta_dot.*t8.*t22.*x_dot.*4.60827495054675e-1+beta_dot.*t10.*t20.*x_dot.*2.13136126875;
et63 = beta_dot.*t10.*t22.*x_dot.*8.034765927723e-1+beta_dot.*t12.*t22.*x_dot.*(2.43e+2./4.0e+1)+beta_dot.*t14.*t20.*x_dot.*1.356463770693052+beta_dot.*t17.*x_dot.*y.*1.113499082493609-gamma_dot.*t11.*t21.*y_dot.*6.571125e-1+gamma_dot.*t19.*x.*x_dot.*2.42733855853125e-2;
et64 = gamma_dot.*t21.*x.*x_dot.*8.920377619816162e-3-gamma_dot.*t16.*y.*y_dot.*1.113499082493609-gamma_dot.*t21.*y.*y_dot.*3.49813839375e-4+t3.*t5.*t6.*t8.*9.11363378203125e-2-t3.*t5.*t7.*t8.*3.79660646334375e-1+t3.*t5.*t6.*t10.*1.82272675640625e-1;
et65 = t3.*t5.*t7.*t10.*1.82272675640625e-1-t2.*t5.*t8.*t14.*8.215338565858331e-1-t2.*t5.*t8.*t16.*1.25953697330909e+1-t2.*t5.*t10.*t14.*6.607430465625e-1-t2.*t5.*t10.*t16.*4.207791216973153e+1;
et66 = t5.*t6.*t8.*t15.*(-3.702668647058184e-1)-t2.*t3.*t11.*t19.*3.2231368125-t5.*t7.*t8.*t15.*1.395238550791759e-1-t5.*t6.*t8.*t17.*1.49538522145242e-1-t5.*t6.*t10.*t15.*1.152881550522619e-1;
et67 = t2.*t3.*t11.*t21.*(-5.0904703125)+t3.*t6.*t8.*t20.*9.229385294181562e-3+t5.*t7.*t10.*t15.*7.520171240086312e-2-t3.*t7.*t8.*t20.*1.395238550791759e-1+t5.*t6.*t10.*t17.*1.021275309790742+t5.*t6.*t12.*t15.*5.1890625e-1;
et68 = t3.*t6.*t8.*t22.*(-8.986136153566162e-3)+t3.*t6.*t10.*t20.*6.009924096961312e-2+t5.*t7.*t12.*t15.*5.1890625e-1+t2.*t8.*t10.*t20.*8.691046875e+1+t3.*t7.*t10.*t20.*7.520171240086312e-2-t5.*t6.*t12.*t17.*5.1890625e-1-t3.*t6.*t10.*t22.*2.522030193384975e-3;
et69 = t3.*t6.*t12.*t20.*5.1890625e-1-t2.*t8.*t10.*t22.*8.691046875e+1+t3.*t7.*t12.*t20.*5.1890625e-1+t3.*t6.*t12.*t22.*6.3736875e-1-t2.*t8.*t14.*t20.*2.389716404930681e+1-t2.*t10.*t14.*t20.*4.568980831862581e+1+t6.*t8.*t11.*t21.*(8.1e+1./3.2e+1)-t2.*t11.*t15.*t19.*5.0904703125-t2.*t12.*t14.*t20.*2.48315625e+1;
et70 = t6.*t8.*t15.*t20.*(-1.585246582988082e-1)+t6.*t11.*t14.*t19.*3.728253949729313+t6.*t10.*t15.*t20.*1.018753279597357+t7.*t11.*t14.*t19.*4.657472815354313-t6.*t11.*t14.*t21.*1.57356813655125e-1;
et71 = t6.*t11.*t16.*t19.*(-4.446644496604313)+t6.*t13.*t14.*t19.*(8.1e+1./3.2e+1)+t6.*t12.*t15.*t20.*1.184625e-1+t7.*t13.*t14.*t19.*(8.1e+1./3.2e+1)-t6.*t13.*t14.*t21.*(8.1e+1./3.2e+1)-t6.*t13.*t16.*t19.*(8.1e+1./3.2e+1)+t3.*t4.*t5.*x.*4.72011110787216e+1+t4.*t5.*t15.*x.*1.734623023299468e+1;
et72 = t3.*t4.*t20.*x.*1.734623023299468e+1+t4.*t11.*t21.*x.*2.48315625e+1-t2.*t3.*t19.*y.*7.06952395454004e-1-t2.*t3.*t21.*y.*7.377287986524673e-1+t6.*t8.*t14.*y.*3.1119725109375+t7.*t8.*t14.*y.*3.1119725109375;
et73 = t6.*t8.*t16.*y.*(-1.934657338925812)+t7.*t8.*t16.*y.*1.143638156386687-t6.*t8.*t18.*y.*1.143638156386687+t6.*t8.*t19.*y.*8.89135003125e-1+t6.*t8.*t21.*y.*3.26753758967625e-1;
et74 = t2.*t15.*t19.*y.*(-7.377287986524673e-1)+t7.*t8.*t21.*y.*8.43058125e-3+t6.*t14.*t19.*y.*5.519842940019625e-1+t7.*t14.*t19.*y.*6.218138900190319e-1;
et75 = t6.*t14.*t21.*y.*(-7.391820761112725e-4)-t6.*t16.*t19.*y.*4.865108980231346e-1+t4.*t16.*x.*y.*1.744191826590139e+1+t4.*t19.*x.*y.*8.72241438065625;
et76 = t4.*t21.*x.*y.*3.205454375472401+T_beta.*t5.*t10.*t14.*x.*(3.15e+2./8.0)+T_gamma.*t3.*t5.*t8.*y.*(3.15e+2./8.0)+beta_dot.*gamma_dot.*t3.*t19.*x.*3.014641757352721+beta_dot.*gamma_dot.*t3.*t21.*x.*1.107869471670417-beta_dot.*gamma_dot.*t10.*t17.*x.*6.735403125e-2;
et77 = beta_dot.*gamma_dot.*t11.*t22.*x.*5.68265625e-1+beta_dot.*gamma_dot.*t15.*t19.*x.*1.107869471670417+T_beta.*t3.*t19.*x.*y.*5.110875+beta_dot.*gamma_dot.*t20.*x.*y.*1.996108082015625e-1+beta_dot.*gamma_dot.*t22.*x.*y.*7.335621888823181e-2+beta_dot.*t5.*t8.*t14.*x_dot.*1.23581941875;
et78 = beta_dot.*t5.*t8.*t16.*x_dot.*5.13572670054675e-1+beta_dot.*t5.*t10.*t16.*x_dot.*1.042899850157805e+1+beta_dot.*t3.*t11.*t21.*x_dot.*1.9024875+beta_dot.*t8.*t10.*t22.*x_dot.*(5.67e+2./1.6e+2)+beta_dot.*t8.*t14.*t20.*x_dot.*9.7440016510935e-1+beta_dot.*t10.*t14.*t20.*x_dot.*1.123247509435035e+1+beta_dot.*t11.*t15.*t19.*x_dot.*1.9024875;
et79 = beta_dot.*t12.*t14.*t20.*x_dot.*(2.43e+2./4.0e+1)-beta_dot.*t3.*t19.*x.*y_dot.*6.6862952235e-2+beta_dot.*t3.*t19.*x_dot.*y.*4.3692906009375e-1-beta_dot.*t3.*t21.*x.*y_dot.*2.45718826743654e-2+beta_dot.*t3.*t21.*x_dot.*y.*1.643995399764465e-1-beta_dot.*t11.*t22.*x.*y_dot.*(8.1e+1./3.2e+1);
et80 = beta_dot.*t15.*t19.*x.*y_dot.*(-2.45718826743654e-2)+beta_dot.*t15.*t19.*x_dot.*y.*1.277898622470056+gamma_dot.*t3.*t5.*t8.*y_dot.*6.223945021875+gamma_dot.*t5.*t8.*t15.*y_dot.*2.287276312773375-gamma_dot.*t5.*t10.*t15.*y_dot.*1.347080625e-1+gamma_dot.*t3.*t8.*t20.*y_dot.*2.287276312773375;
et81 = gamma_dot.*t3.*t10.*t20.*y_dot.*(-1.347080625e-1)-gamma_dot.*t11.*t14.*t19.*y_dot.*6.571125e-1+gamma_dot.*t10.*t21.*x.*x_dot.*6.9103125e-2+gamma_dot.*t14.*t19.*x.*x_dot.*8.920377619816162e-3-beta_dot.*t20.*x.*y.*y_dot.*8.89135003125e-1-beta_dot.*t22.*x.*y.*y_dot.*3.26753758967625e-1-gamma_dot.*t8.*t21.*y.*y_dot.*1.3820625e-1;
et82 = gamma_dot.*t14.*t19.*y.*y_dot.*(-1.113848896332984)+t5.*t6.*t8.*t10.*t15.*5.1890625e-1-t5.*t7.*t8.*t10.*t15.*6.9103125e-2+t5.*t6.*t8.*t10.*t17.*6.9103125e-2+t3.*t6.*t8.*t10.*t20.*5.1890625e-1-t3.*t7.*t8.*t10.*t20.*6.9103125e-2+t3.*t6.*t8.*t10.*t22.*6.9103125e-2-t2.*t8.*t10.*t14.*t20.*8.691046875e+1+t6.*t8.*t11.*t14.*t19.*(8.1e+1./3.2e+1)+t6.*t8.*t10.*t15.*t20.*1.3820625e-1;
et83 = t4.*t5.*t10.*t15.*x.*1.375984701399375e+2+t3.*t4.*t10.*t20.*x.*1.375984701399375e+2+t4.*t11.*t14.*t19.*x.*2.48315625e+1+t2.*t3.*t8.*t19.*y.*1.530362525461875e+2-t2.*t3.*t8.*t21.*y.*2.1206154375e+1-t2.*t8.*t15.*t19.*y.*2.1206154375e+1-t6.*t8.*t14.*t19.*y.*4.718528579958188;
et84 = t7.*t8.*t14.*t19.*y.*1.152068737636687-t6.*t8.*t14.*t21.*y.*2.295706894023375-t6.*t8.*t16.*t19.*y.*3.439345050410062+t4.*t14.*t19.*x.*y.*2.064737264137379e+1-beta_dot.*gamma_dot.*t5.*t14.*x.*y.*1.82272675640625e-1;
et85 = beta_dot.*gamma_dot.*t5.*t16.*x.*y.*1.046996356790246+beta_dot.*gamma_dot.*t14.*t20.*x.*y.*1.120352575678478+beta_dot.*t8.*t10.*t14.*t20.*x_dot.*(5.67e+2./1.6e+2)-beta_dot.*t3.*t8.*t19.*x_dot.*y.*6.9103125e-2+beta_dot.*t3.*t8.*t21.*x_dot.*y.*8.64675e-1-beta_dot.*t3.*t10.*t21.*x.*y_dot.*5.1890625e-1+beta_dot.*t8.*t15.*t19.*x_dot.*y.*8.64675e-1-beta_dot.*t10.*t15.*t19.*x.*y_dot.*5.1890625e-1;
et86 = beta_dot.*t11.*t14.*t20.*x.*y_dot.*(-8.1e+1./3.2e+1)+gamma_dot.*t10.*t14.*t19.*x.*x_dot.*6.9103125e-2-beta_dot.*t5.*t16.*x.*y.*y_dot.*2.470743e-2-beta_dot.*t14.*t20.*x.*y.*y_dot.*3.51461188967625e-1-gamma_dot.*t8.*t14.*t19.*y.*y_dot.*1.3820625e-1+gamma_dot.*t5.*t15.*x.*x_dot.*y.*8.969585625e-3+gamma_dot.*t3.*t20.*x.*x_dot.*y.*8.969585625e-3-beta_dot.*gamma_dot.*t3.*t10.*t19.*x.*1.77827000625;
et87 = beta_dot.*gamma_dot.*t5.*t11.*t16.*x.*(-1.17601875)+beta_dot.*gamma_dot.*t3.*t10.*t21.*x.*8.002540551088125-beta_dot.*gamma_dot.*t3.*t12.*t21.*x.*(8.1e+1./1.6e+1)+beta_dot.*gamma_dot.*t10.*t15.*t19.*x.*7.935186519838125-beta_dot.*gamma_dot.*t11.*t14.*t20.*x.*6.07753125e-1-beta_dot.*gamma_dot.*t12.*t15.*t19.*x.*(8.1e+1./1.6e+1);
et88 = T_gamma.*t14.*2.66889011383505e+1+T_gamma.*t19.*8.3845125e-3+t2.*t20.*3.022661151896329e-2-t2.*t22.*1.61272804021875e-3+T_gamma.*t8.*t14.*(4.41e+2./8.0)+T_gamma.*t8.*t19.*(6.3e+1./4.0)+T_gamma.*t10.*t19.*(6.3e+1./4.0)+T_beta.*t5.*x.*3.07125e-1-T_beta.*t20.*x.*1.9215+beta_dot.*t20.*x_dot.*1.05105853125e-5;
et89 = beta_dot.*t22.*x_dot.*(-6.575853375e-5)+t2.*t5.*t8.*6.7790165625e-1+t2.*t5.*t14.*9.6214901770012e+1-t2.*t5.*t16.*5.133505284707247-t5.*t6.*t15.*2.104341503770595;
et90 = t5.*t6.*t17.*(-8.064242877427253e-1)-t3.*t6.*t20.*6.61094196091875e-4+t2.*t8.*t20.*5.2054137612225e+1-t3.*t6.*t22.*2.533440581098562e-4+t2.*t10.*t20.*5.6779583955975e+1;
et91 = t2.*t10.*t22.*(-3.029450625)-t2.*t14.*t20.*5.135118012747465+t6.*t11.*t19.*1.974375e-2+t7.*t11.*t19.*1.974375e-2-t6.*t11.*t21.*1.23525e-1+t7.*t11.*t21.*3.088125e-1-t6.*t15.*t20.*8.066776318008352e-1;
et92 = t2.*t15.*y.*(-5.890907703762414e+1)+t6.*t14.*y.*3.345644392700366e-2+t7.*t14.*y.*3.345644392700366e-2-t6.*t16.*y.*2.42773682854924e-1+t7.*t16.*y.*5.232930973198009e-1;
et93 = t6.*t18.*y.*9.419275751756416e-1+t6.*t19.*y.*1.05105853125e-5+t7.*t19.*y.*1.05105853125e-5-t6.*t21.*y.*6.575853375e-5+t7.*t21.*y.*1.64396334375e-4-T_beta.*t5.*t14.*x.*1.9215+T_gamma.*t3.*t5.*y.*3.22875+T_beta.*t15.*x.*y.*(4.41e+2./8.0);
et94 = beta_dot.*t5.*t14.*x_dot.*3.345644392700366e-2-beta_dot.*t5.*t16.*x_dot.*2.093172389279204e-1+beta_dot.*t10.*t20.*x_dot.*1.974375e-2-beta_dot.*t10.*t22.*x_dot.*1.23525e-1-beta_dot.*t14.*t20.*x_dot.*2.093829974616704e-1+beta_dot.*t17.*x_dot.*y.*1.201000551225773e+1;
et95 = gamma_dot.*t11.*t21.*y_dot.*(-5.67e+2./8.0e+1)+gamma_dot.*t19.*x.*x_dot.*5.39004375e-4-gamma_dot.*t21.*x.*x_dot.*3.3722325e-3-gamma_dot.*t16.*y.*y_dot.*1.201000551225773e+1-gamma_dot.*t21.*y.*y_dot.*3.773030625e-3+t3.*t5.*t6.*t8.*2.023734375e-3-t3.*t5.*t7.*t8.*8.43058125e-3+t3.*t5.*t6.*t10.*4.04746875e-3;
et96 = t3.*t5.*t7.*t10.*4.04746875e-3+t2.*t5.*t8.*t14.*1.944873129709125e+2-t2.*t5.*t8.*t16.*1.06030771875e+1-t2.*t5.*t10.*t14.*7.1266584375-t5.*t6.*t8.*t15.*4.3675363125-t2.*t3.*t11.*t19.*3.47641875e+1+t5.*t7.*t8.*t15.*5.2745175e-2-t5.*t6.*t8.*t17.*1.612896232691362;
et97 = t5.*t6.*t10.*t15.*(-2.937009375e-2)-t3.*t6.*t8.*t20.*1.2569113125+t5.*t7.*t10.*t15.*6.33065625e-2+t3.*t7.*t8.*t20.*5.2745175e-2+t5.*t6.*t10.*t17.*6.118954568628862-t3.*t6.*t8.*t22.*4.60827495054675e-1-t3.*t6.*t10.*t20.*1.2671638875+t3.*t7.*t10.*t20.*6.33065625e-2;
et98 = t3.*t6.*t10.*t22.*(-4.74011029742175e-1)+t3.*t6.*t12.*t22.*(5.67e+2./1.6e+2)-t2.*t8.*t14.*t20.*1.06030771875e+1-t2.*t10.*t14.*t20.*3.029450625-t6.*t8.*t15.*t20.*2.073723727746038-t6.*t11.*t14.*t19.*1.4326875e-1+t6.*t10.*t15.*t20.*5.644943538886687+t7.*t11.*t14.*t19.*3.088125e-1;
et99 = t6.*t11.*t14.*t21.*1.28233125+t6.*t11.*t16.*t19.*1.28233125+t6.*t12.*t15.*t20.*(5.67e+2./1.6e+2)+t3.*t4.*t5.*x.*1.048127599954012-t4.*t5.*t15.*x.*6.55751626637895-t3.*t4.*t20.*x.*6.55751626637895+t2.*t3.*t19.*y.*1.162130799575925e+1;
et100 = t2.*t3.*t21.*y.*(-6.21037378125e-1)+t6.*t8.*t14.*y.*6.9103125e-2+t7.*t8.*t14.*y.*6.9103125e-2-t6.*t8.*t16.*y.*1.3820625e-1-t7.*t8.*t16.*y.*4.323375e-1+t6.*t8.*t18.*y.*4.323375e-1+t6.*t8.*t19.*y.*1.974375e-2-t6.*t8.*t21.*y.*1.23525e-1-t2.*t15.*t19.*y.*6.21037378125e-1+t7.*t8.*t21.*y.*4.323375e-1;
et101 = t6.*t14.*t19.*y.*(-4.639709668594829e-1)+t7.*t14.*t19.*y.*5.234574936541759e-1-t6.*t14.*t21.*y.*9.726308333433338e-2+t6.*t16.*t19.*y.*8.446644918413082e-1+t4.*t16.*x.*y.*1.881254666584125e+2;
et102 = t4.*t19.*x.*y.*1.936861875e-1-t4.*t21.*x.*y.*1.21178025+beta_dot.*gamma_dot.*t3.*t19.*x.*6.694184008900732e-2-beta_dot.*gamma_dot.*t3.*t21.*x.*4.188156149158407e-1-beta_dot.*gamma_dot.*t10.*t17.*x.*7.2646875e-1-beta_dot.*gamma_dot.*t15.*t19.*x.*4.188156149158407e-1+T_beta.*t3.*t19.*x.*y.*(4.41e+2./8.0);
et103 = beta_dot.*gamma_dot.*t20.*x.*y.*4.432471875e-3-beta_dot.*gamma_dot.*t22.*x.*y.*2.77313625e-2-beta_dot.*t5.*t8.*t14.*x_dot.*6.9103125e-2+beta_dot.*t5.*t8.*t16.*x_dot.*4.323375e-1+beta_dot.*t5.*t10.*t16.*x_dot.*1.4529375+beta_dot.*t3.*t11.*t21.*x_dot.*(5.67e+2./8.0e+1)+beta_dot.*t8.*t14.*t20.*x_dot.*4.323375e-1+beta_dot.*t10.*t14.*t20.*x_dot.*1.3294125+beta_dot.*t11.*t15.*t19.*x_dot.*(5.67e+2./8.0e+1)-beta_dot.*t3.*t19.*x.*y_dot.*1.48473e-3;
et104 = beta_dot.*t3.*t19.*x_dot.*y.*4.04746875e-3+beta_dot.*t3.*t21.*x.*y_dot.*9.28908e-3-beta_dot.*t3.*t21.*x_dot.*y.*2.1549594375e-2+beta_dot.*t15.*t19.*x.*y_dot.*9.28908e-3+beta_dot.*t15.*t19.*x_dot.*y.*1.198845591788272e+1+gamma_dot.*t3.*t5.*t8.*y_dot.*1.3820625e-1-gamma_dot.*t5.*t8.*t15.*y_dot.*8.64675e-1-gamma_dot.*t5.*t10.*t15.*y_dot.*1.4529375-gamma_dot.*t3.*t8.*t20.*y_dot.*8.64675e-1;
et105 = gamma_dot.*t3.*t10.*t20.*y_dot.*(-1.4529375)-gamma_dot.*t11.*t14.*t19.*y_dot.*(5.67e+2./8.0e+1)-gamma_dot.*t14.*t19.*x.*x_dot.*3.3722325e-3-beta_dot.*t20.*x.*y.*y_dot.*1.974375e-2+beta_dot.*t22.*x.*y.*y_dot.*1.23525e-1-gamma_dot.*t8.*t21.*y.*y_dot.*(5.67e+2./8.0e+1)-gamma_dot.*t14.*t19.*y.*y_dot.*1.201377854288273e+1-t5.*t7.*t8.*t10.*t15.*(5.67e+2./1.6e+2)+t5.*t6.*t8.*t10.*t17.*(5.67e+2./1.6e+2)-t3.*t7.*t8.*t10.*t20.*(5.67e+2./1.6e+2);
et106 = t3.*t6.*t8.*t10.*t22.*(5.67e+2./1.6e+2)+t6.*t8.*t10.*t15.*t20.*(5.67e+2./8.0e+1)+t4.*t5.*t10.*t15.*x.*3.47641875e+1+t3.*t4.*t10.*t20.*x.*3.47641875e+1+t2.*t3.*t8.*t19.*y.*8.691046875e+1-t2.*t3.*t8.*t21.*y.*8.691046875e+1-t2.*t8.*t15.*t19.*y.*8.691046875e+1-t6.*t8.*t14.*t19.*y.*2.6173125e-1+t6.*t8.*t14.*t21.*y.*4.323375e-1+t6.*t8.*t16.*t19.*y.*8.64675e-1;
et107 = t4.*t14.*t19.*x.*y.*1.869136864084125e+2-beta_dot.*gamma_dot.*t5.*t14.*x.*y.*4.04746875e-3+beta_dot.*gamma_dot.*t5.*t16.*x.*y.*1.204052469225772e+1+beta_dot.*gamma_dot.*t14.*t20.*x.*y.*1.201279332975773e+1+beta_dot.*t3.*t8.*t21.*x_dot.*y.*(5.67e+2./1.6e+2)-beta_dot.*t3.*t10.*t21.*x.*y_dot.*(5.67e+2./1.6e+2)+beta_dot.*t8.*t15.*t19.*x_dot.*y.*(5.67e+2./1.6e+2)-beta_dot.*t10.*t15.*t19.*x.*y_dot.*(5.67e+2./1.6e+2);
et108 = beta_dot.*t5.*t16.*x.*y.*y_dot.*(-2.6649e-1)-beta_dot.*t14.*t20.*x.*y.*y_dot.*1.42965e-1-gamma_dot.*t8.*t14.*t19.*y.*y_dot.*(5.67e+2./8.0e+1)+gamma_dot.*t5.*t15.*x.*x_dot.*y.*9.6744375e-2+gamma_dot.*t3.*t20.*x.*x_dot.*y.*9.6744375e-2-beta_dot.*gamma_dot.*t3.*t10.*t19.*x.*3.94875e-2-beta_dot.*gamma_dot.*t5.*t11.*t16.*x.*(5.67e+2./8.0e+1)+beta_dot.*gamma_dot.*t3.*t10.*t21.*x.*1.042621875+beta_dot.*gamma_dot.*t10.*t15.*t19.*x.*3.16153125e-1-beta_dot.*gamma_dot.*t11.*t14.*t20.*x.*(5.67e+2./8.0e+1);
plant_model = [x_dot;t51.*(et1+et2+et3+et4+et5+et6+et7+et8+et9+et10+et11+et12+et13+et14+et15+et16+et17+et18+et19+et20+et21+et22+et23+et24+et25+et26+et27+et28+et29+et30+et31+et32+et33+et34+et35);beta_dot;-t51.*(et36+et37+et38+et39+et40+et41+et42+et43+et44+et45+et46+et47+et48+et49+et50+et51);y_dot;t51.*(et52+et53+et54+et55+et56+et57+et58+et59+et60+et61+et62+et63+et64+et65+et66+et67+et68+et69+et70+et71+et72+et73+et74+et75+et76+et77+et78+et79+et80+et81+et82+et83+et84+et85+et86+et87);gamma_dot;t51.*(et88+et89+et90+et91+et92+et93+et94+et95+et96+et97+et98+et99+et100+et101+et102+et103+et104+et105+et106+et107+et108)];

== matlab function Angular_Input_Sliding_Mode/Setpoint_Vectors/x_Setpoint_Function ==
  data: t input; des_traj_sym_x output
function des_traj_sym_x = x_s_vec(t)
%#codegen

%    This function was generated by the Symbolic Math Toolbox version 9.1.
%    03-Nov-2022 15:11:17

t2 = pi.^2;
t3 = t./2.0;
t4 = (t.*pi)./3.0;
t5 = t.*pi.*(2.0./3.0);
t6 = -t3;
t8 = cos(t4);
t9 = cos(t5);
t10 = sin(t4);
t11 = sin(t5);
t7 = exp(t6);
t12 = t7-1.0;
des_traj_sym_x = [t7.*(3.0./2.0e+1)-t8.*t9.*t12.*(3.0./1.0e+1);t7.*(-3.0./4.0e+1)+t7.*t8.*t9.*(3.0./2.0e+1)+(t8.*t11.*t12.*pi)./5.0+(t9.*t10.*t12.*pi)./1.0e+1;t7.*(3.0./8.0e+1)-t7.*t8.*t9.*(3.0./4.0e+1)-(t7.*t8.*t11.*pi)./5.0-(t7.*t9.*t10.*pi)./1.0e+1+(t2.*t8.*t9.*t12)./6.0-t2.*t10.*t11.*t12.*(2.0./1.5e+1)];

== matlab function Angular_Input_Sliding_Mode/Setpoint_Vectors/y_Setpoint_Function ==
  data: t input; des_traj_sym_y output
function des_traj_sym_y = y_s_vec(t)
%#codegen

%    This function was generated by the Symbolic Math Toolbox version 9.1.
%    03-Nov-2022 15:11:17

t2 = pi.^2;
t3 = t./2.0;
t4 = (t.*pi)./3.0;
t5 = t.*pi.*(2.0./3.0);
t6 = -t3;
t8 = cos(t4);
t9 = cos(t5);
t10 = sin(t4);
t11 = sin(t5);
t7 = exp(t6);
t12 = t7-1.0;
des_traj_sym_y = [t7.*(3.0./2.0e+1)-t9.*t10.*t12.*(3.0./1.0e+1);t7.*(-3.0./4.0e+1)+t7.*t9.*t10.*(3.0./2.0e+1)-(t8.*t9.*t12.*pi)./1.0e+1+(t10.*t11.*t12.*pi)./5.0;t7.*(3.0./8.0e+1)-t7.*t9.*t10.*(3.0./4.0e+1)+(t7.*t8.*t9.*pi)./1.0e+1-(t7.*t10.*t11.*pi)./5.0+t2.*t8.*t11.*t12.*(2.0./1.5e+1)+(t2.*t9.*t10.*t12)./6.0];

== matlab function Angular_Input_Sliding_Mode/Controller y dimension/Nullifying Input ==
  data: y input; u_hat_y output; y_dot input; gamma_dot input; gamma_ddot input; y_dot_s input; y_ddot_s input
function u_hat_y = u_hat_y(y,y_dot,gamma_dot,gamma_ddot,y_dot_s,y_ddot_s)
%#codegen

%    This function was generated by the Symbolic Math Toolbox version 9.1.
%    03-Nov-2022 15:11:17

u_hat_y = gamma_ddot.*1.323139653414883e-2+y_dot.*(1.4e+2./9.81e+2)-y_dot_s.*(1.4e+2./9.81e+2)-y_ddot_s.*(1.4e+2./9.81e+2)+gamma_dot.^2.*y.*(1.0e+2./9.81e+2);

== matlab function Angular_Input_Sliding_Mode/beta inner loop/T_hat_beta ==
  data: x input; T_hat_beta output
function T_hat_beta = T_hat_beta(x)
%#codegen

%    This function was generated by the Symbolic Math Toolbox version 9.1.
%    03-Nov-2022 15:11:17

T_hat_beta = x.*(-2.20725);

== matlab function Angular_Input_Sliding_Mode/gamma inner loop/T_hat_gamma ==
  data: y input; T_hat_gamma output
function T_hat_gamma = T_hat_gamma(y)
%#codegen

%    This function was generated by the Symbolic Math Toolbox version 9.1.
%    03-Nov-2022 15:11:17

T_hat_gamma = y.*2.20725;

== matlab function Angular_Input_Sliding_Mode/Controller y dimension/BL Logic ==
  data: S input; port output; S_BL_value parameter
function port = fcn(S,S_BL_value)

if abs(S) <= S_BL_value

    port = 1; %If we are in the boundary layer, use the boundary layer proportional law

else 
    port = 2; %Outside, use the signum law
end

== matlab function Angular_Input_Sliding_Mode/Controller x dimension/Nullifying Input ==
  data: x input; u_hat_x output; x_dot input; beta_dot input; beta_ddot input; x_dot_s input; x_ddot_s input
function u_hat_x = u_hat_x(x,x_dot,beta_dot,beta_ddot,x_dot_s,x_ddot_s)
%#codegen

%    This function was generated by the Symbolic Math Toolbox version 9.1.
%    03-Nov-2022 15:11:17

u_hat_x = beta_ddot.*1.323139653414883e-2-x_dot.*(1.4e+2./9.81e+2)+x_dot_s.*(1.4e+2./9.81e+2)+x_ddot_s.*(1.4e+2./9.81e+2)-beta_dot.^2.*x.*(1.0e+2./9.81e+2);

== matlab function Angular_Input_Sliding_Mode/Controller x dimension/BL Logic ==
  data: S input; port output; S_BL_value parameter
function port = fcn(S,S_BL_value)

if abs(S) <= S_BL_value

    port = 1; %If we are in the boundary layer, use the boundary layer proportional law

else 
    port = 2; %Outside, use the signum law
end
